simulink model "time_gongji_huace"  (R2019b)
settings: Solver=ode3  StartTime=0.0  StopTime=6000  FixedStep=0.01  MaxStep=0.01  RelTol=1e-3
values from neighbouring files (symbols this model uses):
  bias_gyro_z_gongji = -0.7e-3    (= -0.0007)    [sych_ite_KVHpost_daoyuan_huace.m]
  g = 9.8    [sych_ite_KVHpost_daoyuan_huace.m]
settings Model: Creator=luyishi_E480  LastModifiedBy=xie_z
settings DataIOCC: SaveOutput=off  SignalLogging=off  DSMLogging=off  InspectSignalLogs=on  SaveTime=off  ReturnWorkspaceOutputs=off
settings DebuggingCC: InheritedTsInSrcMsg=none

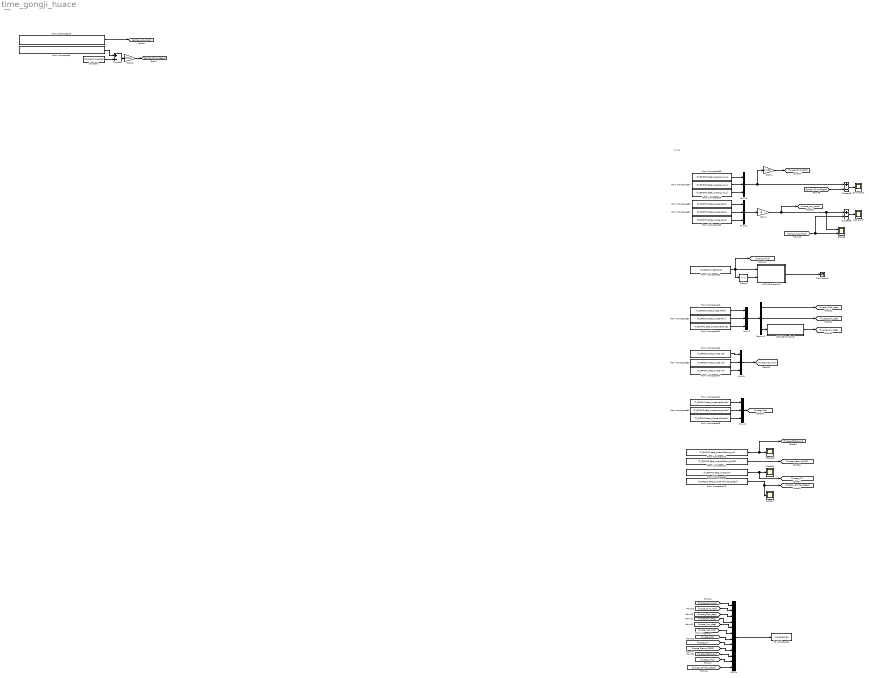
== system time_gongji_huace ==
  note: huace
  note: gongji
  ACC error2 : Scope
  Constant : Constant  Value=bias_gyro_z_gongji
  Delay3 : Delay  DelayLength=1  InitialCondition=0
  Demux2 : Demux  Outputs=3
  From Workspace18 : FromWorkspace  VariableName=[Time,RawData_table.IMU_ACC_x,RawData_table.IMU_ACC_y,RawData_table.IMU_ACC_z]  Interpolate=off  OutputAfterFinalValue=Holding final value
  From Workspace2 : FromWorkspace  VariableName=[Time,RawData_table.IMU_Gyro_x,RawData_table.IMU_Gyro_y,RawData_table.IMU_Gyro_z]  Interpolate=off  OutputAfterFinalValue=Holding final value
  From Workspace53 : FromWorkspace  VariableName=[T_GPCHC,data_huace.acc_z]  Interpolate=off  OutputAfterFinalValue=Holding final value
  From Workspace54 : FromWorkspace  VariableName=[T_GPCHC,data_huace.acc_y]  Interpolate=off  OutputAfterFinalValue=Holding final value
  From Workspace55 : FromWorkspace  VariableName=[T_GPCHC,data_huace.gyro_x]  Interpolate=off  OutputAfterFinalValue=Holding final value
  From Workspace56 : FromWorkspace  VariableName=[T_GPCHC,data_huace.gyro_z]  Interpolate=off  OutputAfterFinalValue=Holding final value
  From Workspace57 : FromWorkspace  VariableName=[T_GPCHC,data_huace.gyro_y]  Interpolate=off  OutputAfterFinalValue=Holding final value
  From Workspace58 : FromWorkspace  VariableName=[T_GPCHC,data_huace.acc_x]  Interpolate=off  OutputAfterFinalValue=Holding final value
  From Workspace59 : FromWorkspace  VariableName=[T_GPCHC,T_GPCHC]  Interpolate=off  OutputAfterFinalValue=Holding final value
  From Workspace60 : FromWorkspace  VariableName=[T_GPCHC,data_huace.Roll]  Interpolate=off  OutputAfterFinalValue=Holding final value
  From Workspace61 : FromWorkspace  VariableName=[T_GPCHC,data_huace.Heading]  Interpolate=off  OutputAfterFinalValue=Holding final value
  From Workspace62 : FromWorkspace  VariableName=[T_GPCHC,data_huace.Pitch]  Interpolate=off  OutputAfterFinalValue=Holding final value
  From Workspace63 : FromWorkspace  VariableName=[T_GPCHC,data_huace.VE]  Interpolate=off  OutputAfterFinalValue=Holding final value
  From Workspace64 : FromWorkspace  VariableName=[T_GPCHC,data_huace.VU]  Interpolate=off  OutputAfterFinalValue=Holding final value
  From Workspace65 : FromWorkspace  VariableName=[T_GPCHC,data_huace.VN]  Interpolate=off  OutputAfterFinalValue=Holding final value
  From Workspace66 : FromWorkspace  VariableName=[T_GPCHC,data_huace.Longitude]  Interpolate=off  OutputAfterFinalValue=Holding final value
  From Workspace67 : FromWorkspace  VariableName=[T_GPCHC,data_huace.Lattitude]  Interpolate=off  OutputAfterFinalValue=Holding final value
  From Workspace68 : FromWorkspace  VariableName=[T_GPCHC,data_huace.Altitude]  Interpolate=off  OutputAfterFinalValue=Holding final value
  From Workspace69 : FromWorkspace  VariableName=[T_GPCHC,data_huace.SV]  Interpolate=off  OutputAfterFinalValue=Holding final value
  From Workspace70 : FromWorkspace  VariableName=[T_GPCHC,data_huace.vehicle_speed]  Interpolate=off  OutputAfterFinalValue=Holding final value
  From Workspace71 : FromWorkspace  VariableName=[T_GPCHC,data_huace.Status_GNSS]  Interpolate=off  OutputAfterFinalValue=Holding final value
  From Workspace72 : FromWorkspace  VariableName=[T_GPCHC,data_huace.Status_sys]  Interpolate=off  OutputAfterFinalValue=Holding final value
  Gain1 : Gain  Gain=pi/180
  Gain4 : Gain  Gain=g
  Gain6 : Gain  Gain=180/pi
  Gyro error2 : Scope
  MATLAB Function4 : MATLAB Function  TreatAsAtomicUnit=on
  MATLAB Function5 : MATLAB Function  TreatAsAtomicUnit=on
  Mux14 : Mux  Inputs=12
  Mux{15..16,18..20} (5 alike) : Mux  Inputs=3
  Scope10 : Scope
  Scope6 : Scope  NumInputPorts=2
  Scope7 : Scope
  Scope9 : Scope
  Subtract : Sum  Inputs=+-
  Subtract3 : Sum  Inputs=+-
  Subtract6 : Sum  Inputs=+-
  Terminator2 : Terminator
  To Workspace2 : ToWorkspace  VariableName=huace_gongji  SaveFormat=Structure With Time  SampleTime=-1
  wires:
  Subtract/1 -> Gain6/1
  Constant/1 -> Subtract/2
  From Workspace2/1 -> Subtract/1  "gongji"
  From Workspace18/1 -> [gongji_Acc_mpss]  "gongji"
  Gain6/1 -> [gongji_Gyro_degps]  "gongji"
  [huace_Acc_mpss] -> Mux14/1
  [huace_SV] -> Mux14/8
  [huace_Time] -> Mux14/11
  [huace_Yaw_deg] -> Mux14/5
  [huace_vehicle_speed] -> Mux14/12
  Mux14/1 -> To Workspace2/1
  [huace_Roll_deg] -> Mux14/4
  [huace_Pitch_deg] -> Mux14/3
  [huace_Pos] -> Mux14/7
  [huace_Status_GNSS] -> Mux14/9
  [huace_Vel_mps] -> Mux14/6
  [huace_Gyro_rdps] -> Mux14/2
  [huace_Status_sys] -> Mux14/10
  From Workspace57/1 -> Mux16/2
  From Workspace53/1 -> Mux15/3
  Subtract6/1 -> ACC error2/1
  [gongji_Gyro_degps] -> Subtract3/2  "gongji"
  Gain4/1 -> [huace_Acc_mpss], Scope6/1, Subtract6/1  "huace"
  Gain1/1 -> [huace_Gyro_rdps]
  From Workspace55/1 -> Mux16/1
  From Workspace54/1 -> Mux15/2
  From Workspace56/1 -> Mux16/3
  From Workspace58/1 -> Mux15/1
  [gongji_Acc_mpss] -> Subtract6/2, Scope6/2  "gongji"
  Mux15/1 -> Gain4/1  "KVH"
  Mux16/1 -> Subtract3/1, Gain1/1  "huace"
  Subtract3/1 -> Gyro error2/1
  MATLAB Function4/1(y) -> Terminator2/1
  From Workspace59/1 -> [huace_Time], Delay3/1, MATLAB Function4/1(x)
  Delay3/1 -> MATLAB Function4/2(x_k_1)
  From Workspace60/1 -> Mux18/2
  From Workspace62/1 -> Mux18/1
  MATLAB Function5/1(Heading_ENU) -> [huace_Yaw_deg]
  Demux2/1 -> [huace_Pitch_deg]
  Demux2/2 -> [huace_Roll_deg]
  Mux18/1 -> Demux2/1
  Demux2/3 -> MATLAB Function5/1(Heading_North)
  From Workspace61/1 -> Mux18/3
  From Workspace63/1 -> Mux19/1
  From Workspace64/1 -> Mux19/3
  From Workspace65/1 -> Mux19/2
  Mux19/1 -> [huace_Vel_mps]
  Mux20/1 -> [huace_Pos]
  From Workspace68/1 -> Mux20/3
  From Workspace66/1 -> Mux20/2
  From Workspace67/1 -> Mux20/1
  From Workspace70/1 -> Scope7/1, [huace_vehicle_speed]
  From Workspace71/1 -> [huace_Status_GNSS]
  From Workspace69/1 -> [huace_SV], Scope9/1
  From Workspace72/1 -> Scope10/1, [huace_Status_sys]

== matlab function time_gongji_huace/MATLAB Function4 ==
  data: y output; x input; x_k_1 input
function y  = fcn(x,x_k_1)
    if x ~= x_k_1
        y = uint8(1);
    else
        y = uint8(0);
    end
end

== matlab function time_gongji_huace/MATLAB Function5 ==
  data: Heading_North input; Heading_ENU output size=1
function Heading_ENU = fcn(Heading_North)
% Heading_ENU:以北为零顺时针为正0-360°
% Heading_North:以北为零逆时针为正-180-180°

% Heading_North = Heading_North + 0.5 + 3.8;
if Heading_North <= 180
    Heading_ENU = 0 - Heading_North;
else
    Heading_ENU = 360 - Heading_North;
end
